simulink model "tst4_20211106"  (R2013b)
settings: Solver=VariableStepDiscrete  StartTime=0.0  StopTime=StopTime  RelTol=1e-3
values from neighbouring files (symbols this model uses):
  a2 = a(2)    [design_2ord_sc_sigma_delta_adc_20211008.m]    (also in run_limited_bit_width_sum.m; run_limited_bit_width_sum_enob.m; run_tst1.m)
  amp = umax    [design_2ord_sc_sigma_delta_adc_20211008.m]    (also in run_limited_bit_width_sum.m; run_limited_bit_width_sum_enob.m = 0.8; run_tst1.m = 0.01)
  b1 = b(1)    [design_2ord_sc_sigma_delta_adc_20211008.m]    (also in run_limited_bit_width_sum.m; run_limited_bit_width_sum_enob.m; run_tst1.m)
  c1 = c(1)    [design_2ord_sc_sigma_delta_adc_20211008.m]    (also in run_limited_bit_width_sum.m; run_limited_bit_width_sum_enob.m; run_tst1.m)
  den = 2^(cic_order*log(osr)/log(2))    [design_2ord_sc_sigma_delta_adc_20211008.m]    (also in run_limited_bit_width_sum.m; run_limited_bit_width_sum_enob.m; run_tst1.m)
  fin = fs*7/128/osr    (= 0.213623046875)    [design_2ord_sc_sigma_delta_adc_20211008.m]    (also in run_limited_bit_width_sum.m = 54.6875; run_limited_bit_width_sum_enob.m; run_tst1.m = 54.6875)
  fs = 256e3    (= 256000)    [design_2ord_sc_sigma_delta_adc_20211008.m]    (also in run_limited_bit_width_sum.m; run_limited_bit_width_sum_enob.m; run_tst1.m)
  osr = 2^16    (= 65536)    [cal_c1_20211015.m]    (also in design_2ord_sc_sigma_delta_adc_20211008.m; run_limited_bit_width_sum.m = 256; run_limited_bit_width_sum_enob.m; run_tst1.m = 256)
  vos = 10e-3    (= 0.01)    [design_2ord_sc_sigma_delta_adc_20211008.m]    (also in run_limited_bit_width_sum.m; run_limited_bit_width_sum_enob.m)
settings Model: Creator=eric  LastModifiedBy=eric

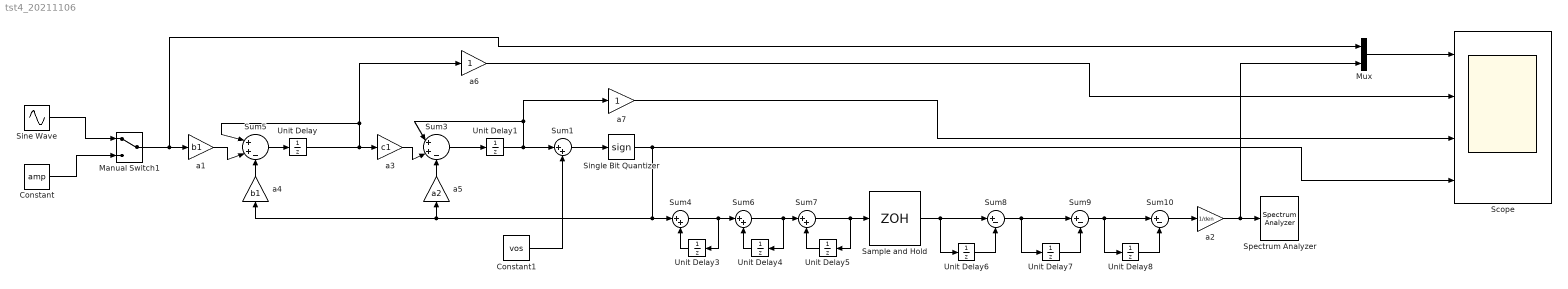
== system tst4_20211106 ==
  Constant : Constant  Value=amp  SampleTime=1/fs
  Constant1 : Constant  Value=vos  SampleTime=1/fs
  Manual Switch1 : ManualSwitch
  Mux : Mux  Inputs=2
  Sample and Hold : ZeroOrderHold  SampleTime=osr/fs
  Scope : Scope  NumInputPorts=4
      settings: TimeRange=0.09  YMin=0.00999~-0.2~-0.2~-1.5  YMax=0.01001~0.6~0.2~1.5  MaxDataPoints=20000
  Sine Wave : Sin  Amplitude=amp  Frequency=2*pi*fin  SampleTime=1/fs
  Single Bit Quantizer : Signum  SampleTime=1/fs
  Spectrum Analyzer : SpectrumAnalyzer
      settings: CopyFcn=scopeextensions.ScopeBlock.onCoreBlockCopy(gcbh);  DeleteFcn=scopeextensions.ScopeBlock.callback(gcbh, 'onBlockDelete');  PreSaveFcn=scopeextensions.ScopeBlock.callback(gcbh, 'onModelSave');  NameChangeFcn=scopeextensions.ScopeBlock.callback(gcbh, 'onBlockRename');  DestroyFcn=scopeextensions.ScopeBlock.onBlockDestroy(gcbh)  CloseFcn=scopeextensions.ScopeBlock.callback(gcbh, 'onBlockClose');  PreDeleteFcn=scopeextensions.ScopeBlock.callback(gcbh, 'onBlockPreDelete');
  Sum{1,4,6..7} (4 alike) : Sum  Inputs=|++  AccumDataTypeStr=double  SampleTime=1/fs
  Sum10 : Sum  Inputs=|+-  AccumDataTypeStr=double  SampleTime=osr/fs
  Sum3 : Sum  Inputs=|++-  AccumDataTypeStr=double  SampleTime=1/fs
  Sum5 : Sum  Inputs=|++-  AccumDataTypeStr=double  SampleTime=1/fs
  Sum8 : Sum  Inputs=|+-  AccumDataTypeStr=double  SampleTime=osr/fs
  Sum9 : Sum  Inputs=|+-  AccumDataTypeStr=double  SampleTime=osr/fs
  Unit Delay{,1,3..5} (5 alike) : UnitDelay  SampleTime=1/fs
  Unit Delay6 : UnitDelay  SampleTime=osr/fs
  Unit Delay7 : UnitDelay  SampleTime=osr/fs
  Unit Delay8 : UnitDelay  SampleTime=osr/fs
  a1 : Gain  Gain=b1  SampleTime=1/fs
  a2 : Gain  Gain=1/den  SampleTime=osr/fs
  a3 : Gain  Gain=c1  SampleTime=1/fs
  a4 : Gain  Gain=b1  SampleTime=1/fs
  a5 : Gain  Gain=a2  SampleTime=1/fs
  a6 : Gain  SampleTime=1/fs
  a7 : Gain  SampleTime=1/fs
  wires:
  Sum3/1 -> Unit Delay1/1
  Sum5/1 -> Unit Delay/1
  Unit Delay3/1 -> Sum4/2
  Sum4/1 -> Sum6/1, Unit Delay3/1
  Unit Delay4/1 -> Sum6/2
  Sum6/1 -> Unit Delay4/1, Sum7/1
  Unit Delay5/1 -> Sum7/2
  Sum7/1 -> Unit Delay5/1, Sample and Hold/1
  Sample and Hold/1 -> Unit Delay6/1, Sum8/1
  Unit Delay6/1 -> Sum8/2
  Unit Delay7/1 -> Sum9/2
  Sum8/1 -> Unit Delay7/1, Sum9/1
  Sum9/1 -> Unit Delay8/1, Sum10/1
  Unit Delay8/1 -> Sum10/2
  Sum10/1 -> a2/1
  a2/1 -> Spectrum Analyzer/1, Mux/2
  Manual Switch1/1 -> Mux/1, a1/1
  Sine Wave/1 -> Manual Switch1/1
  Constant/1 -> Manual Switch1/2
  Mux/1 -> Scope/1
  a4/1 -> Sum5/3
  a1/1 -> Sum5/2
  Unit Delay/1 -> a6/1, Sum5/1, a3/1
  a5/1 -> Sum3/3
  a3/1 -> Sum3/2
  Unit Delay1/1 -> Sum1/1, a7/1, Sum3/1
  a7/1 -> Scope/3
  a6/1 -> Scope/2
  Single Bit Quantizer/1 -> a5/1, a4/1, Sum4/1, Scope/4
  Sum1/1 -> Single Bit Quantizer/1
  Constant1/1 -> Sum1/2
